simulink model "ALL_JP360_DBW_V6_5_1103"  (R2022a)
settings: Solver=FixedStepAuto  StartTime=0.0  StopTime=inf  FixedStep=0.01  RelTol=1e-3  EnableMultiTasking=on
model workspace (MAT data in the model file):
  g = 9.8
undefined symbols (not defined in the file or in its folder): canChannel, delta_v_p, IPM_Line_C0, IPM_Line_C1, IPM_Line_C2, IPM_Line_C3, M, M_p, MRR_ObjDistX, MRR_ObjDistY, MRR_ObjFusionCamID, MRR_ObjFusionSig, MRR_ObjID, MRR_ObjRelVelX, MRR_ObjRelVelY, MRR_ObjType, MRR_ObjUpdFlg, none, obj_vaild, untracktime, V, videoinput
libraries: canfdmsglib x230, canfdlib x76, slpidlib x24, simulink x18, dspstat3 x14, ctrlSharedLib x1, simulink_extras x1, imaqlib x1, realtime_pacer_lib x1, dspvision x1, visionsinks x1
(part 7 of 55)

== system ALL_JP360_DBW_V6_5_1103/MsgFromCAN/Subsystem ==
  VR_ADCU_MRR_Obj_01_02_0x690FromOutData : Inport
  VR_ADCU_MRR_Obj_03_04_0x691FromOutData : Inport  Port=2
  VR_ADCU_MRR_Obj_05_06_0x692FromOutData : Inport  Port=3
  VR_ADCU_MRR_Obj_07_08_0x693FromOutData : Inport  Port=4
  VR_ADCU_MRR_Obj_09_10_0x694FromOutData : Inport  Port=5
  VR_ADCU_MRR_Obj_11_12_0x695FromOutData : Inport  Port=6
  VR_ADCU_MRR_Obj_13_14_0x696FromOutData : Inport  Port=7
  VR_ADCU_MRR_Obj_15_16_0x697FromOutData : Inport  Port=8
  VR_ADCU_MRR_Obj_17_18_0x698FromOutData : Inport  Port=9
  VR_ADCU_MRR_Obj_19_20_0x699FromOutData : Inport  Port=10
  VR_ADCU_MRR_Obj_21_22_0x69AFromOutData : Inport  Port=11
  VR_ADCU_MRR_Obj_23_24_0x69BFromOutData : Inport  Port=12
  VR_ADCU_MRR_Obj_25_26_0x69CFromOutData : Inport  Port=13
  VR_ADCU_MRR_Obj_27_28_0x69DFromOutData : Inport  Port=14
  VR_ADCU_MRR_Obj_29_30_0x69EFromOutData : Inport  Port=15
  VR_ADCU_MRR_Obj_31_32_0x69FFromOutData : Inport  Port=16
  Subsystem1 : Subsystem
  Subsystem10 : Subsystem
  Subsystem11 : Subsystem
  Subsystem12 : Subsystem
  Subsystem13 : Subsystem
  Subsystem14 : Subsystem
  Subsystem15 : Subsystem
  Subsystem16 : Subsystem
  Subsystem2 : Subsystem
  Subsystem3 : Subsystem
  Subsystem4 : Subsystem
  Subsystem5 : Subsystem
  Subsystem6 : Subsystem
  Subsystem7 : Subsystem
  Subsystem8 : Subsystem
  Subsystem9 : Subsystem
  1 : Outport
  2 : Outport  Port=2
  3 : Outport  Port=3
  4 : Outport  Port=4
  5 : Outport  Port=5
  6 : Outport  Port=6
  7 : Outport  Port=7
  8 : Outport  Port=8
  9 : Outport  Port=9
  10 : Outport  Port=10
  11 : Outport  Port=11
  12 : Outport  Port=12
  13 : Outport  Port=13
  14 : Outport  Port=14
  15 : Outport  Port=15
  16 : Outport  Port=16
  17 : Outport  Port=17
  18 : Outport  Port=18
  19 : Outport  Port=19
  20 : Outport  Port=20
  21 : Outport  Port=21
  22 : Outport  Port=22
  23 : Outport  Port=23
  24 : Outport  Port=24
  25 : Outport  Port=25
  26 : Outport  Port=26
  27 : Outport  Port=27
  28 : Outport  Port=28
  29 : Outport  Port=29
  30 : Outport  Port=30
  31 : Outport  Port=31
  32 : Outport  Port=32
  wires:
  VR_ADCU_MRR_Obj_01_02_0x690FromOutData/1 -> Subsystem16/1(VR_ADCU_MRR_ObjHeader_0x680FromOutData)  "VR_ADCU_MRR_ObjHeader_0x680FromOutData"
  Subsystem16/1(Out1) -> 1/1
  Subsystem16/2(Out2) -> 2/1
  Subsystem1/2(Out2) -> 4/1
  Subsystem1/1(Out1) -> 3/1
  VR_ADCU_MRR_Obj_03_04_0x691FromOutData/1 -> Subsystem1/1(VR_ADCU_MRR_ObjHeader_0x680FromOutData)  "VR_ADCU_MRR_ObjHeader_0x680FromOutData"
  Subsystem3/1(Out1) -> 7/1
  Subsystem3/2(Out2) -> 8/1
  Subsystem2/2(Out2) -> 6/1
  Subsystem2/1(Out1) -> 5/1
  VR_ADCU_MRR_Obj_05_06_0x692FromOutData/1 -> Subsystem2/1(VR_ADCU_MRR_ObjHeader_0x680FromOutData)
  VR_ADCU_MRR_Obj_07_08_0x693FromOutData/1 -> Subsystem3/1(VR_ADCU_MRR_ObjHeader_0x680FromOutData)
  Subsystem6/1(Out1) -> 13/1
  Subsystem6/2(Out2) -> 14/1
  Subsystem7/2(Out2) -> 16/1
  Subsystem7/1(Out1) -> 15/1
  Subsystem5/1(Out1) -> 11/1
  Subsystem5/2(Out2) -> 12/1
  Subsystem4/2(Out2) -> 10/1
  Subsystem4/1(Out1) -> 9/1
  Subsystem12/1(Out1) -> 25/1
  Subsystem12/2(Out2) -> 26/1
  Subsystem13/2(Out2) -> 28/1
  Subsystem13/1(Out1) -> 27/1
  Subsystem15/1(Out1) -> 31/1
  Subsystem15/2(Out2) -> 32/1
  Subsystem14/2(Out2) -> 30/1
  Subsystem14/1(Out1) -> 29/1
  Subsystem10/1(Out1) -> 21/1
  Subsystem10/2(Out2) -> 22/1
  Subsystem11/2(Out2) -> 24/1
  Subsystem11/1(Out1) -> 23/1
  Subsystem9/1(Out1) -> 19/1
  Subsystem9/2(Out2) -> 20/1
  Subsystem8/2(Out2) -> 18/1
  Subsystem8/1(Out1) -> 17/1
  VR_ADCU_MRR_Obj_09_10_0x694FromOutData/1 -> Subsystem4/1(VR_ADCU_MRR_ObjHeader_0x680FromOutData)
  VR_ADCU_MRR_Obj_11_12_0x695FromOutData/1 -> Subsystem5/1(VR_ADCU_MRR_ObjHeader_0x680FromOutData)
  VR_ADCU_MRR_Obj_13_14_0x696FromOutData/1 -> Subsystem6/1(VR_ADCU_MRR_ObjHeader_0x680FromOutData)
  VR_ADCU_MRR_Obj_15_16_0x697FromOutData/1 -> Subsystem7/1(VR_ADCU_MRR_ObjHeader_0x680FromOutData)
  VR_ADCU_MRR_Obj_17_18_0x698FromOutData/1 -> Subsystem8/1(VR_ADCU_MRR_ObjHeader_0x680FromOutData)
  VR_ADCU_MRR_Obj_19_20_0x699FromOutData/1 -> Subsystem9/1(VR_ADCU_MRR_ObjHeader_0x680FromOutData)
  VR_ADCU_MRR_Obj_21_22_0x69AFromOutData/1 -> Subsystem10/1(VR_ADCU_MRR_ObjHeader_0x680FromOutData)
  VR_ADCU_MRR_Obj_23_24_0x69BFromOutData/1 -> Subsystem11/1(VR_ADCU_MRR_ObjHeader_0x680FromOutData)
  VR_ADCU_MRR_Obj_25_26_0x69CFromOutData/1 -> Subsystem12/1(VR_ADCU_MRR_ObjHeader_0x680FromOutData)
  VR_ADCU_MRR_Obj_27_28_0x69DFromOutData/1 -> Subsystem13/1(VR_ADCU_MRR_ObjHeader_0x680FromOutData)
  VR_ADCU_MRR_Obj_29_30_0x69EFromOutData/1 -> Subsystem14/1(VR_ADCU_MRR_ObjHeader_0x680FromOutData)
  VR_ADCU_MRR_Obj_31_32_0x69FFromOutData/1 -> Subsystem15/1(VR_ADCU_MRR_ObjHeader_0x680FromOutData)

== system ALL_JP360_DBW_V6_5_1103/MsgFromCAN/Subsystem1 ==
  VR_ADCU_IPM_Obj_01_0x650FromOutData : Inport
  VR_ADCU_IPM_Obj_02_0x651FromOutData : Inport  Port=2
  VR_ADCU_IPM_Obj_03_0x652FromOutData : Inport  Port=3
  VR_ADCU_IPM_Obj_04_0x653FromOutData : Inport  Port=4
  VR_ADCU_IPM_Obj_05_0x654FromOutData : Inport  Port=5
  VR_ADCU_IPM_Obj_06_0x655FromOutData : Inport  Port=6
  VR_ADCU_IPM_Obj_07_0x656FromOutData : Inport  Port=7
  VR_ADCU_IPM_Obj_08_0x657FromOutData : Inport  Port=8
  VR_ADCU_IPM_Obj_09_0x658FromOutData : Inport  Port=9
  VR_ADCU_IPM_Obj_10_0x659FromOutData : Inport  Port=10
  VR_ADCU_IPM_Obj_11_0x65AFromOutData : Inport  Port=11
  VR_ADCU_IPM_Obj_12_0x65BFromOutData : Inport  Port=12
  VR_ADCU_IPM_Obj_13_0x65CFromOutData : Inport  Port=13
  VR_ADCU_IPM_Obj_14_0x65DFromOutData : Inport  Port=14
  VR_ADCU_IPM_Obj_15_0x65EFromOutData : Inport  Port=15
  VR_ADCU_IPM_Obj_16_0x65FFromOutData : Inport  Port=16
  VR_ADCU_IPM_Obj_17_0x660FromOutData : Inport  Port=17
  VR_ADCU_IPM_Obj_18_0x661FromOutData : Inport  Port=18
  VR_ADCU_IPM_Obj_19_0x662FromOutData : Inport  Port=19
  VR_ADCU_IPM_Obj_20_0x663FromOutData : Inport  Port=20
  Subsystem1 : Subsystem
  Subsystem10 : Subsystem
  Subsystem11 : Subsystem
  Subsystem12 : Subsystem
  Subsystem13 : Subsystem
  Subsystem14 : Subsystem
  Subsystem15 : Subsystem
  Subsystem16 : Subsystem
  Subsystem17 : Subsystem
  Subsystem18 : Subsystem
  Subsystem19 : Subsystem
  Subsystem2 : Subsystem
  Subsystem20 : Subsystem
  Subsystem3 : Subsystem
  Subsystem4 : Subsystem
  Subsystem5 : Subsystem
  Subsystem6 : Subsystem
  Subsystem7 : Subsystem
  Subsystem8 : Subsystem
  Subsystem9 : Subsystem
  1 : Outport
  2 : Outport  Port=2
  3 : Outport  Port=3
  4 : Outport  Port=4
  5 : Outport  Port=5
  6 : Outport  Port=6
  7 : Outport  Port=7
  8 : Outport  Port=8
  9 : Outport  Port=9
  10 : Outport  Port=10
  11 : Outport  Port=11
  12 : Outport  Port=12
  13 : Outport  Port=13
  14 : Outport  Port=14
  15 : Outport  Port=15
  16 : Outport  Port=16
  17 : Outport  Port=17
  18 : Outport  Port=18
  19 : Outport  Port=19
  20 : Outport  Port=20
  wires:
  VR_ADCU_IPM_Obj_01_0x650FromOutData/1 -> Subsystem7/1(VR_ADCU_MRR_ObjHeader_0x680FromOutData)
  Subsystem7/1(Out2) -> 1/1
  Subsystem1/1(Out2) -> 2/1
  Subsystem2/1(Out2) -> 3/1
  Subsystem3/1(Out2) -> 5/1
  Subsystem5/1(Out2) -> 4/1
  Subsystem4/1(Out2) -> 6/1
  Subsystem9/1(Out2) -> 7/1
  Subsystem6/1(Out2) -> 8/1
  Subsystem8/1(Out2) -> 9/1
  Subsystem10/1(Out2) -> 11/1
  Subsystem16/1(Out2) -> 10/1
  Subsystem15/1(Out2) -> 17/1
  Subsystem18/1(Out2) -> 16/1
  Subsystem17/1(Out2) -> 18/1
  Subsystem11/1(Out2) -> 12/1
  Subsystem12/1(Out2) -> 14/1
  Subsystem14/1(Out2) -> 13/1
  Subsystem13/1(Out2) -> 15/1
  Subsystem20/1(Out2) -> 20/1
  Subsystem19/1(Out2) -> 19/1
  VR_ADCU_IPM_Obj_02_0x651FromOutData/1 -> Subsystem1/1(VR_ADCU_MRR_ObjHeader_0x680FromOutData)
  VR_ADCU_IPM_Obj_03_0x652FromOutData/1 -> Subsystem2/1(VR_ADCU_MRR_ObjHeader_0x680FromOutData)
  VR_ADCU_IPM_Obj_04_0x653FromOutData/1 -> Subsystem5/1(VR_ADCU_MRR_ObjHeader_0x680FromOutData)
  VR_ADCU_IPM_Obj_05_0x654FromOutData/1 -> Subsystem3/1(VR_ADCU_MRR_ObjHeader_0x680FromOutData)
  VR_ADCU_IPM_Obj_06_0x655FromOutData/1 -> Subsystem4/1(VR_ADCU_MRR_ObjHeader_0x680FromOutData)
  VR_ADCU_IPM_Obj_07_0x656FromOutData/1 -> Subsystem9/1(VR_ADCU_MRR_ObjHeader_0x680FromOutData)
  VR_ADCU_IPM_Obj_08_0x657FromOutData/1 -> Subsystem6/1(VR_ADCU_MRR_ObjHeader_0x680FromOutData)
  VR_ADCU_IPM_Obj_09_0x658FromOutData/1 -> Subsystem8/1(VR_ADCU_MRR_ObjHeader_0x680FromOutData)
  VR_ADCU_IPM_Obj_10_0x659FromOutData/1 -> Subsystem16/1(VR_ADCU_MRR_ObjHeader_0x680FromOutData)
  VR_ADCU_IPM_Obj_11_0x65AFromOutData/1 -> Subsystem10/1(VR_ADCU_MRR_ObjHeader_0x680FromOutData)
  VR_ADCU_IPM_Obj_12_0x65BFromOutData/1 -> Subsystem11/1(VR_ADCU_MRR_ObjHeader_0x680FromOutData)
  VR_ADCU_IPM_Obj_13_0x65CFromOutData/1 -> Subsystem14/1(VR_ADCU_MRR_ObjHeader_0x680FromOutData)
  VR_ADCU_IPM_Obj_14_0x65DFromOutData/1 -> Subsystem12/1(VR_ADCU_MRR_ObjHeader_0x680FromOutData)
  VR_ADCU_IPM_Obj_15_0x65EFromOutData/1 -> Subsystem13/1(VR_ADCU_MRR_ObjHeader_0x680FromOutData)
  VR_ADCU_IPM_Obj_16_0x65FFromOutData/1 -> Subsystem18/1(VR_ADCU_MRR_ObjHeader_0x680FromOutData)
  VR_ADCU_IPM_Obj_17_0x660FromOutData/1 -> Subsystem15/1(VR_ADCU_MRR_ObjHeader_0x680FromOutData)
  VR_ADCU_IPM_Obj_18_0x661FromOutData/1 -> Subsystem17/1(VR_ADCU_MRR_ObjHeader_0x680FromOutData)
  VR_ADCU_IPM_Obj_19_0x662FromOutData/1 -> Subsystem19/1(VR_ADCU_MRR_ObjHeader_0x680FromOutData)
  VR_ADCU_IPM_Obj_20_0x663FromOutData/1 -> Subsystem20/1(VR_ADCU_MRR_ObjHeader_0x680FromOutData)

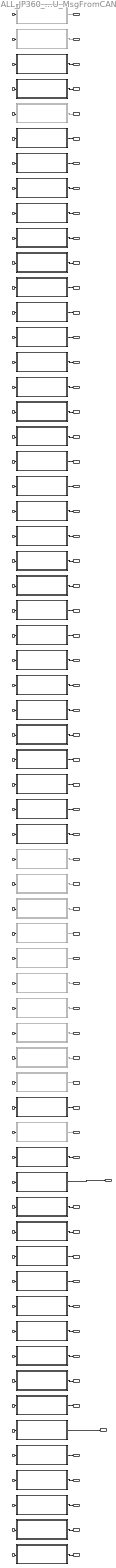
== system ALL_JP360_DBW_V6_5_1103/MsgFromCAN/VR_ADCU_MsgFromCAN ==
  VR_ADCU_IPM_0x345FromInData : Inport  OutDataTypeStr=Bus:CAN_FD_MESSAGE_BUS
  VR_ADCU_IPM_0x347FromInData : Inport  Port=2  OutDataTypeStr=Bus:CAN_FD_MESSAGE_BUS
  VR_ADCU_IPM_LeftLine_0x378FromInData : Inport  Port=3  OutDataTypeStr=Bus:CAN_FD_MESSAGE_BUS
  VR_ADCU_IPM_LeftLine_0x380FromInData : Inport  Port=4  OutDataTypeStr=Bus:CAN_FD_MESSAGE_BUS
  VR_ADCU_IPM_LineHeader_0x631FromInData : Inport  Port=5  OutDataTypeStr=Bus:CAN_FD_MESSAGE_BUS
  VR_ADCU_IPM_Line_01_0x640FromInData : Inport  Port=6  OutDataTypeStr=Bus:CAN_FD_MESSAGE_BUS
  VR_ADCU_IPM_Line_02_0x641FromInData : Inport  Port=7  OutDataTypeStr=Bus:CAN_FD_MESSAGE_BUS
  VR_ADCU_IPM_Line_03_0x642FromInData : Inport  Port=8  OutDataTypeStr=Bus:CAN_FD_MESSAGE_BUS
  VR_ADCU_IPM_Line_04_0x643FromInData : Inport  Port=9  OutDataTypeStr=Bus:CAN_FD_MESSAGE_BUS
  VR_ADCU_IPM_Line_05_0x644FromInData : Inport  Port=10  OutDataTypeStr=Bus:CAN_FD_MESSAGE_BUS
  VR_ADCU_IPM_Line_06_0x645FromInData : Inport  Port=11  OutDataTypeStr=Bus:CAN_FD_MESSAGE_BUS
  VR_ADCU_IPM_ObjHeader_0x630FromInData : Inport  Port=12  OutDataTypeStr=Bus:CAN_FD_MESSAGE_BUS
  VR_ADCU_IPM_Obj_01_0x650FromInData : Inport  Port=13  OutDataTypeStr=Bus:CAN_FD_MESSAGE_BUS
  VR_ADCU_IPM_Obj_02_0x651FromInData : Inport  Port=14  OutDataTypeStr=Bus:CAN_FD_MESSAGE_BUS
  VR_ADCU_IPM_Obj_03_0x652FromInData : Inport  Port=15  OutDataTypeStr=Bus:CAN_FD_MESSAGE_BUS
  VR_ADCU_IPM_Obj_04_0x653FromInData : Inport  Port=16  OutDataTypeStr=Bus:CAN_FD_MESSAGE_BUS
  VR_ADCU_IPM_Obj_05_0x654FromInData : Inport  Port=17  OutDataTypeStr=Bus:CAN_FD_MESSAGE_BUS
  VR_ADCU_IPM_Obj_06_0x655FromInData : Inport  Port=18  OutDataTypeStr=Bus:CAN_FD_MESSAGE_BUS
  VR_ADCU_IPM_Obj_07_0x656FromInData : Inport  Port=19  OutDataTypeStr=Bus:CAN_FD_MESSAGE_BUS
  VR_ADCU_IPM_Obj_08_0x657FromInData : Inport  Port=20  OutDataTypeStr=Bus:CAN_FD_MESSAGE_BUS
  VR_ADCU_IPM_Obj_09_0x658FromInData : Inport  Port=21  OutDataTypeStr=Bus:CAN_FD_MESSAGE_BUS
  VR_ADCU_IPM_Obj_10_0x659FromInData : Inport  Port=22  OutDataTypeStr=Bus:CAN_FD_MESSAGE_BUS
  VR_ADCU_IPM_Obj_11_0x65AFromInData : Inport  Port=23  OutDataTypeStr=Bus:CAN_FD_MESSAGE_BUS
  VR_ADCU_IPM_Obj_12_0x65BFromInData : Inport  Port=24  OutDataTypeStr=Bus:CAN_FD_MESSAGE_BUS
  VR_ADCU_IPM_Obj_13_0x65CFromInData : Inport  Port=25  OutDataTypeStr=Bus:CAN_FD_MESSAGE_BUS
  VR_ADCU_IPM_Obj_14_0x65DFromInData : Inport  Port=26  OutDataTypeStr=Bus:CAN_FD_MESSAGE_BUS
  VR_ADCU_IPM_Obj_15_0x65EFromInData : Inport  Port=27  OutDataTypeStr=Bus:CAN_FD_MESSAGE_BUS
  VR_ADCU_IPM_Obj_16_0x65FFromInData : Inport  Port=28  OutDataTypeStr=Bus:CAN_FD_MESSAGE_BUS
  VR_ADCU_IPM_Obj_17_0x660FromInData : Inport  Port=29  OutDataTypeStr=Bus:CAN_FD_MESSAGE_BUS
  VR_ADCU_IPM_Obj_18_0x661FromInData : Inport  Port=30  OutDataTypeStr=Bus:CAN_FD_MESSAGE_BUS
  VR_ADCU_IPM_Obj_19_0x662FromInData : Inport  Port=31  OutDataTypeStr=Bus:CAN_FD_MESSAGE_BUS
  VR_ADCU_IPM_Obj_20_0x663FromInData : Inport  Port=32  OutDataTypeStr=Bus:CAN_FD_MESSAGE_BUS
  VR_ADCU_IPM_RightLine_0x590FromInData : Inport  Port=33  OutDataTypeStr=Bus:CAN_FD_MESSAGE_BUS
  VR_ADCU_IPM_RightLine_0x591FromInData : Inport  Port=34  OutDataTypeStr=Bus:CAN_FD_MESSAGE_BUS
  VR_ADCU_IPM_Traffic_01_0x670FromInData : Inport  Port=35  OutDataTypeStr=Bus:CAN_FD_MESSAGE_BUS
  VR_ADCU_IPM_Traffic_02_0x671FromInData : Inport  Port=36  OutDataTypeStr=Bus:CAN_FD_MESSAGE_BUS
  VR_ADCU_IPM_Traffic_03_0x672FromInData : Inport  Port=37  OutDataTypeStr=Bus:CAN_FD_MESSAGE_BUS
  VR_ADCU_IPM_Traffic_04_0x673FromInData : Inport  Port=38  OutDataTypeStr=Bus:CAN_FD_MESSAGE_BUS
  VR_ADCU_IPM_Traffic_05_0x674FromInData : Inport  Port=39  OutDataTypeStr=Bus:CAN_FD_MESSAGE_BUS
  VR_ADCU_IPM_Traffic_06_0x675FromInData : Inport  Port=40  OutDataTypeStr=Bus:CAN_FD_MESSAGE_BUS
  VR_ADCU_IPM_VLC_0x393FromInData : Inport  Port=41  OutDataTypeStr=Bus:CAN_FD_MESSAGE_BUS
  VR_ADCU_MRR_0x338FromInData : Inport  Port=42  OutDataTypeStr=Bus:CAN_FD_MESSAGE_BUS
  VR_ADCU_MRR_0x339FromInData : Inport  Port=43  OutDataTypeStr=Bus:CAN_FD_MESSAGE_BUS
  VR_ADCU_MRR_0x346FromInData : Inport  Port=44  OutDataTypeStr=Bus:CAN_FD_MESSAGE_BUS
  VR_ADCU_MRR_FRObj_0x379FromInData : Inport  Port=45  OutDataTypeStr=Bus:CAN_FD_MESSAGE_BUS
  VR_ADCU_MRR_LRObj_0x580FromInData : Inport  Port=46  OutDataTypeStr=Bus:CAN_FD_MESSAGE_BUS
  VR_ADCU_MRR_ObjHeader_0x680FromInData : Inport  Port=47  OutDataTypeStr=Bus:CAN_FD_MESSAGE_BUS
  VR_ADCU_MRR_Obj_01_02_0x690FromInData : Inport  Port=48  OutDataTypeStr=Bus:CAN_FD_MESSAGE_BUS
  VR_ADCU_MRR_Obj_03_04_0x691FromInData : Inport  Port=49  OutDataTypeStr=Bus:CAN_FD_MESSAGE_BUS
  VR_ADCU_MRR_Obj_05_06_0x692FromInData : Inport  Port=50  OutDataTypeStr=Bus:CAN_FD_MESSAGE_BUS
  VR_ADCU_MRR_Obj_07_08_0x693FromInData : Inport  Port=51  OutDataTypeStr=Bus:CAN_FD_MESSAGE_BUS
  VR_ADCU_MRR_Obj_09_10_0x694FromInData : Inport  Port=52  OutDataTypeStr=Bus:CAN_FD_MESSAGE_BUS
  VR_ADCU_MRR_Obj_11_12_0x695FromInData : Inport  Port=53  OutDataTypeStr=Bus:CAN_FD_MESSAGE_BUS
  VR_ADCU_MRR_Obj_13_14_0x696FromInData : Inport  Port=54  OutDataTypeStr=Bus:CAN_FD_MESSAGE_BUS
  VR_ADCU_MRR_Obj_15_16_0x697FromInData : Inport  Port=55  OutDataTypeStr=Bus:CAN_FD_MESSAGE_BUS
  VR_ADCU_MRR_Obj_17_18_0x698FromInData : Inport  Port=56  OutDataTypeStr=Bus:CAN_FD_MESSAGE_BUS
  VR_ADCU_MRR_Obj_19_20_0x699FromInData : Inport  Port=57  OutDataTypeStr=Bus:CAN_FD_MESSAGE_BUS
  VR_ADCU_MRR_Obj_21_22_0x69AFromInData : Inport  Port=58  OutDataTypeStr=Bus:CAN_FD_MESSAGE_BUS
  VR_ADCU_MRR_Obj_23_24_0x69BFromInData : Inport  Port=59  OutDataTypeStr=Bus:CAN_FD_MESSAGE_BUS
  VR_ADCU_MRR_Obj_25_26_0x69CFromInData : Inport  Port=60  OutDataTypeStr=Bus:CAN_FD_MESSAGE_BUS
  VR_ADCU_MRR_Obj_27_28_0x69DFromInData : Inport  Port=61  OutDataTypeStr=Bus:CAN_FD_MESSAGE_BUS
  VR_ADCU_MRR_Obj_29_30_0x69EFromInData : Inport  Port=62  OutDataTypeStr=Bus:CAN_FD_MESSAGE_BUS
  VR_ADCU_MRR_Obj_31_32_0x69FFromInData : Inport  Port=63  OutDataTypeStr=Bus:CAN_FD_MESSAGE_BUS
  VR_ADCU_IPM_0x345 : Subsystem  Commented=on  TreatAsAtomicUnit=on
  VR_ADCU_IPM_0x347 : Subsystem  Commented=on  TreatAsAtomicUnit=on
  VR_ADCU_IPM_LeftLine_0x378 : Subsystem  TreatAsAtomicUnit=on
  VR_ADCU_IPM_LeftLine_0x380 : Subsystem  TreatAsAtomicUnit=on
  VR_ADCU_IPM_LineHeader_0x631 : Subsystem  Commented=on  TreatAsAtomicUnit=on
  VR_ADCU_IPM_Line_01_0x640 : Subsystem  TreatAsAtomicUnit=on
  VR_ADCU_IPM_Line_02_0x641 : Subsystem  TreatAsAtomicUnit=on
  VR_ADCU_IPM_Line_03_0x642 : Subsystem  TreatAsAtomicUnit=on
  VR_ADCU_IPM_Line_04_0x643 : Subsystem  TreatAsAtomicUnit=on
  VR_ADCU_IPM_Line_05_0x644 : Subsystem  TreatAsAtomicUnit=on
  VR_ADCU_IPM_Line_06_0x645 : Subsystem  TreatAsAtomicUnit=on
  VR_ADCU_IPM_ObjHeader_0x630 : Subsystem  TreatAsAtomicUnit=on
  VR_ADCU_IPM_Obj_01_0x650 : Subsystem  TreatAsAtomicUnit=on
  VR_ADCU_IPM_Obj_02_0x651 : Subsystem  TreatAsAtomicUnit=on
  VR_ADCU_IPM_Obj_03_0x652 : Subsystem  TreatAsAtomicUnit=on
  VR_ADCU_IPM_Obj_04_0x653 : Subsystem  TreatAsAtomicUnit=on
  VR_ADCU_IPM_Obj_05_0x654 : Subsystem  TreatAsAtomicUnit=on
  VR_ADCU_IPM_Obj_06_0x655 : Subsystem  TreatAsAtomicUnit=on
  VR_ADCU_IPM_Obj_07_0x656 : Subsystem  TreatAsAtomicUnit=on
  VR_ADCU_IPM_Obj_08_0x657 : Subsystem  TreatAsAtomicUnit=on
  VR_ADCU_IPM_Obj_09_0x658 : Subsystem  TreatAsAtomicUnit=on
  VR_ADCU_IPM_Obj_10_0x659 : Subsystem  TreatAsAtomicUnit=on
  VR_ADCU_IPM_Obj_11_0x65A : Subsystem  TreatAsAtomicUnit=on
  VR_ADCU_IPM_Obj_12_0x65B : Subsystem  TreatAsAtomicUnit=on
  VR_ADCU_IPM_Obj_13_0x65C : Subsystem  TreatAsAtomicUnit=on
  VR_ADCU_IPM_Obj_14_0x65D : Subsystem  TreatAsAtomicUnit=on
  VR_ADCU_IPM_Obj_15_0x65E : Subsystem  TreatAsAtomicUnit=on
  VR_ADCU_IPM_Obj_16_0x65F : Subsystem  TreatAsAtomicUnit=on
  VR_ADCU_IPM_Obj_17_0x660 : Subsystem  TreatAsAtomicUnit=on
  VR_ADCU_IPM_Obj_18_0x661 : Subsystem  TreatAsAtomicUnit=on
  VR_ADCU_IPM_Obj_19_0x662 : Subsystem  TreatAsAtomicUnit=on
  VR_ADCU_IPM_Obj_20_0x663 : Subsystem  TreatAsAtomicUnit=on
  VR_ADCU_IPM_RightLine_0x590 : Subsystem  TreatAsAtomicUnit=on
  VR_ADCU_IPM_RightLine_0x591 : Subsystem  TreatAsAtomicUnit=on
  VR_ADCU_IPM_Traffic_01_0x670 : Subsystem  Commented=on  TreatAsAtomicUnit=on
  VR_ADCU_IPM_Traffic_02_0x671 : Subsystem  Commented=on  TreatAsAtomicUnit=on
  VR_ADCU_IPM_Traffic_03_0x672 : Subsystem  Commented=on  TreatAsAtomicUnit=on
  VR_ADCU_IPM_Traffic_04_0x673 : Subsystem  Commented=on  TreatAsAtomicUnit=on
  VR_ADCU_IPM_Traffic_05_0x674 : Subsystem  Commented=on  TreatAsAtomicUnit=on
  VR_ADCU_IPM_Traffic_06_0x675 : Subsystem  Commented=on  TreatAsAtomicUnit=on
  VR_ADCU_IPM_VLC_0x393 : Subsystem  Commented=on  TreatAsAtomicUnit=on
  VR_ADCU_MRR_0x338 : Subsystem  Commented=on  TreatAsAtomicUnit=on
  VR_ADCU_MRR_0x339 : Subsystem  Commented=on  TreatAsAtomicUnit=on
  VR_ADCU_MRR_0x346 : Subsystem  Commented=on  TreatAsAtomicUnit=on
  VR_ADCU_MRR_FRObj_0x379 : Subsystem  TreatAsAtomicUnit=on
  VR_ADCU_MRR_LRObj_0x580 : Subsystem  Commented=on  TreatAsAtomicUnit=on
  VR_ADCU_MRR_ObjHeader_0x680 : Subsystem  TreatAsAtomicUnit=on
  VR_ADCU_MRR_Obj_01_02_0x690 : Subsystem  TreatAsAtomicUnit=on
  VR_ADCU_MRR_Obj_03_04_0x691 : Subsystem  TreatAsAtomicUnit=on
  VR_ADCU_MRR_Obj_05_06_0x692 : Subsystem  TreatAsAtomicUnit=on
  VR_ADCU_MRR_Obj_07_08_0x693 : Subsystem  TreatAsAtomicUnit=on
  VR_ADCU_MRR_Obj_09_10_0x694 : Subsystem  TreatAsAtomicUnit=on
  VR_ADCU_MRR_Obj_11_12_0x695 : Subsystem  TreatAsAtomicUnit=on
  VR_ADCU_MRR_Obj_13_14_0x696 : Subsystem  TreatAsAtomicUnit=on
  VR_ADCU_MRR_Obj_15_16_0x697 : Subsystem  TreatAsAtomicUnit=on
  VR_ADCU_MRR_Obj_17_18_0x698 : Subsystem  TreatAsAtomicUnit=on
  VR_ADCU_MRR_Obj_19_20_0x699 : Subsystem  TreatAsAtomicUnit=on
  VR_ADCU_MRR_Obj_21_22_0x69A : Subsystem  TreatAsAtomicUnit=on
  VR_ADCU_MRR_Obj_23_24_0x69B : Subsystem  TreatAsAtomicUnit=on
  VR_ADCU_MRR_Obj_25_26_0x69C : Subsystem  TreatAsAtomicUnit=on
  VR_ADCU_MRR_Obj_27_28_0x69D : Subsystem  TreatAsAtomicUnit=on
  VR_ADCU_MRR_Obj_29_30_0x69E : Subsystem  TreatAsAtomicUnit=on
  VR_ADCU_MRR_Obj_31_32_0x69F : Subsystem  TreatAsAtomicUnit=on
  VR_ADCU_IPM_0x345FromOutData : Outport  OutDataTypeStr=Bus:VR_ADCU_IPM_0x345
  VR_ADCU_IPM_0x347FromOutData : Outport  Port=2  OutDataTypeStr=Bus:VR_ADCU_IPM_0x347
  VR_ADCU_IPM_LeftLine_0x378FromOutData : Outport  Port=3  OutDataTypeStr=Bus:VR_ADCU_IPM_LeftLine_0x378
  VR_ADCU_IPM_LeftLine_0x380FromOutData : Outport  Port=4  OutDataTypeStr=Bus:VR_ADCU_IPM_LeftLine_0x380
  VR_ADCU_IPM_LineHeader_0x631FromOutData : Outport  Port=5  OutDataTypeStr=Bus:VR_ADCU_IPM_LineHeader_0x631
  VR_ADCU_IPM_Line_01_0x640FromOutData : Outport  Port=6  OutDataTypeStr=Bus:VR_ADCU_IPM_Line_01_0x640
  VR_ADCU_IPM_Line_02_0x641FromOutData : Outport  Port=7  OutDataTypeStr=Bus:VR_ADCU_IPM_Line_02_0x641
  VR_ADCU_IPM_Line_03_0x642FromOutData : Outport  Port=8  OutDataTypeStr=Bus:VR_ADCU_IPM_Line_03_0x642
  VR_ADCU_IPM_Line_04_0x643FromOutData : Outport  Port=9  OutDataTypeStr=Bus:VR_ADCU_IPM_Line_04_0x643
  VR_ADCU_IPM_Line_05_0x644FromOutData : Outport  Port=10  OutDataTypeStr=Bus:VR_ADCU_IPM_Line_05_0x644
  VR_ADCU_IPM_Line_06_0x645FromOutData : Outport  Port=11  OutDataTypeStr=Bus:VR_ADCU_IPM_Line_06_0x645
  VR_ADCU_IPM_ObjHeader_0x630FromOutData : Outport  Port=12  OutDataTypeStr=Bus:VR_ADCU_IPM_ObjHeader_0x630
  VR_ADCU_IPM_Obj_01_0x650FromOutData : Outport  Port=13  OutDataTypeStr=Bus:VR_ADCU_IPM_Obj_01_0x650
  VR_ADCU_IPM_Obj_02_0x651FromOutData : Outport  Port=14  OutDataTypeStr=Bus:VR_ADCU_IPM_Obj_02_0x651
  VR_ADCU_IPM_Obj_03_0x652FromOutData : Outport  Port=15  OutDataTypeStr=Bus:VR_ADCU_IPM_Obj_03_0x652
  VR_ADCU_IPM_Obj_04_0x653FromOutData : Outport  Port=16  OutDataTypeStr=Bus:VR_ADCU_IPM_Obj_04_0x653
  VR_ADCU_IPM_Obj_05_0x654FromOutData : Outport  Port=17  OutDataTypeStr=Bus:VR_ADCU_IPM_Obj_05_0x654
  VR_ADCU_IPM_Obj_06_0x655FromOutData : Outport  Port=18  OutDataTypeStr=Bus:VR_ADCU_IPM_Obj_06_0x655
  VR_ADCU_IPM_Obj_07_0x656FromOutData : Outport  Port=19  OutDataTypeStr=Bus:VR_ADCU_IPM_Obj_07_0x656
  VR_ADCU_IPM_Obj_08_0x657FromOutData : Outport  Port=20  OutDataTypeStr=Bus:VR_ADCU_IPM_Obj_08_0x657
  VR_ADCU_IPM_Obj_09_0x658FromOutData : Outport  Port=21  OutDataTypeStr=Bus:VR_ADCU_IPM_Obj_09_0x658
  VR_ADCU_IPM_Obj_10_0x659FromOutData : Outport  Port=22  OutDataTypeStr=Bus:VR_ADCU_IPM_Obj_10_0x659
  VR_ADCU_IPM_Obj_11_0x65AFromOutData : Outport  Port=23  OutDataTypeStr=Bus:VR_ADCU_IPM_Obj_11_0x65A
  VR_ADCU_IPM_Obj_12_0x65BFromOutData : Outport  Port=24  OutDataTypeStr=Bus:VR_ADCU_IPM_Obj_12_0x65B
  VR_ADCU_IPM_Obj_13_0x65CFromOutData : Outport  Port=25  OutDataTypeStr=Bus:VR_ADCU_IPM_Obj_13_0x65C
  VR_ADCU_IPM_Obj_14_0x65DFromOutData : Outport  Port=26  OutDataTypeStr=Bus:VR_ADCU_IPM_Obj_14_0x65D
  VR_ADCU_IPM_Obj_15_0x65EFromOutData : Outport  Port=27  OutDataTypeStr=Bus:VR_ADCU_IPM_Obj_15_0x65E
  VR_ADCU_IPM_Obj_16_0x65FFromOutData : Outport  Port=28  OutDataTypeStr=Bus:VR_ADCU_IPM_Obj_16_0x65F
  VR_ADCU_IPM_Obj_17_0x660FromOutData : Outport  Port=29  OutDataTypeStr=Bus:VR_ADCU_IPM_Obj_17_0x660
  VR_ADCU_IPM_Obj_18_0x661FromOutData : Outport  Port=30  OutDataTypeStr=Bus:VR_ADCU_IPM_Obj_18_0x661
  VR_ADCU_IPM_Obj_19_0x662FromOutData : Outport  Port=31  OutDataTypeStr=Bus:VR_ADCU_IPM_Obj_19_0x662
  VR_ADCU_IPM_Obj_20_0x663FromOutData : Outport  Port=32  OutDataTypeStr=Bus:VR_ADCU_IPM_Obj_20_0x663
  VR_ADCU_IPM_RightLine_0x590FromOutData : Outport  Port=33  OutDataTypeStr=Bus:VR_ADCU_IPM_RightLine_0x590
  VR_ADCU_IPM_RightLine_0x591FromOutData : Outport  Port=34  OutDataTypeStr=Bus:VR_ADCU_IPM_RightLine_0x591
  VR_ADCU_IPM_Traffic_01_0x670FromOutData : Outport  Port=35  OutDataTypeStr=Bus:VR_ADCU_IPM_Traffic_01_0x670
  VR_ADCU_IPM_Traffic_02_0x671FromOutData : Outport  Port=36  OutDataTypeStr=Bus:VR_ADCU_IPM_Traffic_02_0x671
  VR_ADCU_IPM_Traffic_03_0x672FromOutData : Outport  Port=37  OutDataTypeStr=Bus:VR_ADCU_IPM_Traffic_03_0x672
  VR_ADCU_IPM_Traffic_04_0x673FromOutData : Outport  Port=38  OutDataTypeStr=Bus:VR_ADCU_IPM_Traffic_04_0x673
  VR_ADCU_IPM_Traffic_05_0x674FromOutData : Outport  Port=39  OutDataTypeStr=Bus:VR_ADCU_IPM_Traffic_05_0x674
  VR_ADCU_IPM_Traffic_06_0x675FromOutData : Outport  Port=40  OutDataTypeStr=Bus:VR_ADCU_IPM_Traffic_06_0x675
  VR_ADCU_IPM_VLC_0x393FromOutData : Outport  Port=41  OutDataTypeStr=Bus:VR_ADCU_IPM_VLC_0x393
  VR_ADCU_MRR_0x338FromOutData : Outport  Port=42  OutDataTypeStr=Bus:VR_ADCU_MRR_0x338
  VR_ADCU_MRR_0x339FromOutData : Outport  Port=43  OutDataTypeStr=Bus:VR_ADCU_MRR_0x339
  VR_ADCU_MRR_0x346FromOutData : Outport  Port=44  OutDataTypeStr=Bus:VR_ADCU_MRR_0x346
  VR_ADCU_MRR_FRObj_0x379FromOutData : Outport  Port=45  OutDataTypeStr=Bus:VR_ADCU_MRR_FRObj_0x379
  VR_ADCU_MRR_LRObj_0x580FromOutData : Outport  Port=46  OutDataTypeStr=Bus:VR_ADCU_MRR_LRObj_0x580
  VR_ADCU_MRR_ObjHeader_0x680FromOutData : Outport  Port=47  OutDataTypeStr=Bus:VR_ADCU_MRR_ObjHeader_0x680
  VR_ADCU_MRR_Obj_01_02_0x690FromOutData : Outport  Port=48  OutDataTypeStr=Bus:VR_ADCU_MRR_Obj_01_02_0x690
  VR_ADCU_MRR_Obj_03_04_0x691FromOutData : Outport  Port=49  OutDataTypeStr=Bus:VR_ADCU_MRR_Obj_03_04_0x691
  VR_ADCU_MRR_Obj_05_06_0x692FromOutData : Outport  Port=50  OutDataTypeStr=Bus:VR_ADCU_MRR_Obj_05_06_0x692
  VR_ADCU_MRR_Obj_07_08_0x693FromOutData : Outport  Port=51  OutDataTypeStr=Bus:VR_ADCU_MRR_Obj_07_08_0x693
  VR_ADCU_MRR_Obj_09_10_0x694FromOutData : Outport  Port=52  OutDataTypeStr=Bus:VR_ADCU_MRR_Obj_09_10_0x694
  VR_ADCU_MRR_Obj_11_12_0x695FromOutData : Outport  Port=53  OutDataTypeStr=Bus:VR_ADCU_MRR_Obj_11_12_0x695
  VR_ADCU_MRR_Obj_13_14_0x696FromOutData : Outport  Port=54  OutDataTypeStr=Bus:VR_ADCU_MRR_Obj_13_14_0x696
  VR_ADCU_MRR_Obj_15_16_0x697FromOutData : Outport  Port=55  OutDataTypeStr=Bus:VR_ADCU_MRR_Obj_15_16_0x697
  VR_ADCU_MRR_Obj_17_18_0x698FromOutData : Outport  Port=56  OutDataTypeStr=Bus:VR_ADCU_MRR_Obj_17_18_0x698
  VR_ADCU_MRR_Obj_19_20_0x699FromOutData : Outport  Port=57  OutDataTypeStr=Bus:VR_ADCU_MRR_Obj_19_20_0x699
  VR_ADCU_MRR_Obj_21_22_0x69AFromOutData : Outport  Port=58  OutDataTypeStr=Bus:VR_ADCU_MRR_Obj_21_22_0x69A
  VR_ADCU_MRR_Obj_23_24_0x69BFromOutData : Outport  Port=59  OutDataTypeStr=Bus:VR_ADCU_MRR_Obj_23_24_0x69B
  VR_ADCU_MRR_Obj_25_26_0x69CFromOutData : Outport  Port=60  OutDataTypeStr=Bus:VR_ADCU_MRR_Obj_25_26_0x69C
  VR_ADCU_MRR_Obj_27_28_0x69DFromOutData : Outport  Port=61  OutDataTypeStr=Bus:VR_ADCU_MRR_Obj_27_28_0x69D
  VR_ADCU_MRR_Obj_29_30_0x69EFromOutData : Outport  Port=62  OutDataTypeStr=Bus:VR_ADCU_MRR_Obj_29_30_0x69E
  VR_ADCU_MRR_Obj_31_32_0x69FFromOutData : Outport  Port=63  OutDataTypeStr=Bus:VR_ADCU_MRR_Obj_31_32_0x69F
  wires:
  VR_ADCU_IPM_0x345/1(VR_ADCU_IPM_0x345FromOutData) -> VR_ADCU_IPM_0x345FromOutData/1  "VR_ADCU_IPM_0x345FromOutData"
  VR_ADCU_IPM_0x345FromInData/1 -> VR_ADCU_IPM_0x345/1(VR_ADCU_IPM_0x345FromInData)  "VR_ADCU_IPM_0x345FromInData"
  VR_ADCU_IPM_0x347/1(VR_ADCU_IPM_0x347FromOutData) -> VR_ADCU_IPM_0x347FromOutData/1  "VR_ADCU_IPM_0x347FromOutData"
  VR_ADCU_IPM_0x347FromInData/1 -> VR_ADCU_IPM_0x347/1(VR_ADCU_IPM_0x347FromInData)  "VR_ADCU_IPM_0x347FromInData"
  VR_ADCU_IPM_LeftLine_0x378/1(VR_ADCU_IPM_LeftLine_0x378FromOutData) -> VR_ADCU_IPM_LeftLine_0x378FromOutData/1  "VR_ADCU_IPM_LeftLine_0x378FromOutData"
  VR_ADCU_IPM_LeftLine_0x378FromInData/1 -> VR_ADCU_IPM_LeftLine_0x378/1(VR_ADCU_IPM_LeftLine_0x378FromInData)  "VR_ADCU_IPM_LeftLine_0x378FromInData"
  VR_ADCU_IPM_LeftLine_0x380/1(VR_ADCU_IPM_LeftLine_0x380FromOutData) -> VR_ADCU_IPM_LeftLine_0x380FromOutData/1  "VR_ADCU_IPM_LeftLine_0x380FromOutData"
  VR_ADCU_IPM_LeftLine_0x380FromInData/1 -> VR_ADCU_IPM_LeftLine_0x380/1(VR_ADCU_IPM_LeftLine_0x380FromInData)  "VR_ADCU_IPM_LeftLine_0x380FromInData"
  VR_ADCU_IPM_LineHeader_0x631/1(VR_ADCU_IPM_LineHeader_0x631FromOutData) -> VR_ADCU_IPM_LineHeader_0x631FromOutData/1  "VR_ADCU_IPM_LineHeader_0x631FromOutData"
  VR_ADCU_IPM_LineHeader_0x631FromInData/1 -> VR_ADCU_IPM_LineHeader_0x631/1(VR_ADCU_IPM_LineHeader_0x631FromInData)  "VR_ADCU_IPM_LineHeader_0x631FromInData"
  VR_ADCU_IPM_Line_01_0x640/1(VR_ADCU_IPM_Line_01_0x640FromOutData) -> VR_ADCU_IPM_Line_01_0x640FromOutData/1  "VR_ADCU_IPM_Line_01_0x640FromOutData"
  VR_ADCU_IPM_Line_01_0x640FromInData/1 -> VR_ADCU_IPM_Line_01_0x640/1(VR_ADCU_IPM_Line_01_0x640FromInData)  "VR_ADCU_IPM_Line_01_0x640FromInData"
  VR_ADCU_IPM_Line_02_0x641/1(VR_ADCU_IPM_Line_02_0x641FromOutData) -> VR_ADCU_IPM_Line_02_0x641FromOutData/1  "VR_ADCU_IPM_Line_02_0x641FromOutData"
  VR_ADCU_IPM_Line_02_0x641FromInData/1 -> VR_ADCU_IPM_Line_02_0x641/1(VR_ADCU_IPM_Line_02_0x641FromInData)  "VR_ADCU_IPM_Line_02_0x641FromInData"
  VR_ADCU_IPM_Line_03_0x642/1(VR_ADCU_IPM_Line_03_0x642FromOutData) -> VR_ADCU_IPM_Line_03_0x642FromOutData/1  "VR_ADCU_IPM_Line_03_0x642FromOutData"
  VR_ADCU_IPM_Line_03_0x642FromInData/1 -> VR_ADCU_IPM_Line_03_0x642/1(VR_ADCU_IPM_Line_03_0x642FromInData)  "VR_ADCU_IPM_Line_03_0x642FromInData"
  VR_ADCU_IPM_Line_04_0x643/1(VR_ADCU_IPM_Line_04_0x643FromOutData) -> VR_ADCU_IPM_Line_04_0x643FromOutData/1  "VR_ADCU_IPM_Line_04_0x643FromOutData"
  VR_ADCU_IPM_Line_04_0x643FromInData/1 -> VR_ADCU_IPM_Line_04_0x643/1(VR_ADCU_IPM_Line_04_0x643FromInData)  "VR_ADCU_IPM_Line_04_0x643FromInData"
  VR_ADCU_IPM_Line_05_0x644/1(VR_ADCU_IPM_Line_05_0x644FromOutData) -> VR_ADCU_IPM_Line_05_0x644FromOutData/1  "VR_ADCU_IPM_Line_05_0x644FromOutData"
  VR_ADCU_IPM_Line_05_0x644FromInData/1 -> VR_ADCU_IPM_Line_05_0x644/1(VR_ADCU_IPM_Line_05_0x644FromInData)  "VR_ADCU_IPM_Line_05_0x644FromInData"
  VR_ADCU_IPM_Line_06_0x645/1(VR_ADCU_IPM_Line_06_0x645FromOutData) -> VR_ADCU_IPM_Line_06_0x645FromOutData/1  "VR_ADCU_IPM_Line_06_0x645FromOutData"
  VR_ADCU_IPM_Line_06_0x645FromInData/1 -> VR_ADCU_IPM_Line_06_0x645/1(VR_ADCU_IPM_Line_06_0x645FromInData)  "VR_ADCU_IPM_Line_06_0x645FromInData"
  VR_ADCU_IPM_ObjHeader_0x630/1(VR_ADCU_IPM_ObjHeader_0x630FromOutData) -> VR_ADCU_IPM_ObjHeader_0x630FromOutData/1  "VR_ADCU_IPM_ObjHeader_0x630FromOutData"
  VR_ADCU_IPM_ObjHeader_0x630FromInData/1 -> VR_ADCU_IPM_ObjHeader_0x630/1(VR_ADCU_IPM_ObjHeader_0x630FromInData)  "VR_ADCU_IPM_ObjHeader_0x630FromInData"
  VR_ADCU_IPM_Obj_01_0x650/1(VR_ADCU_IPM_Obj_01_0x650FromOutData) -> VR_ADCU_IPM_Obj_01_0x650FromOutData/1  "VR_ADCU_IPM_Obj_01_0x650FromOutData"
  VR_ADCU_IPM_Obj_01_0x650FromInData/1 -> VR_ADCU_IPM_Obj_01_0x650/1(VR_ADCU_IPM_Obj_01_0x650FromInData)  "VR_ADCU_IPM_Obj_01_0x650FromInData"
  VR_ADCU_IPM_Obj_02_0x651/1(VR_ADCU_IPM_Obj_02_0x651FromOutData) -> VR_ADCU_IPM_Obj_02_0x651FromOutData/1  "VR_ADCU_IPM_Obj_02_0x651FromOutData"
  VR_ADCU_IPM_Obj_02_0x651FromInData/1 -> VR_ADCU_IPM_Obj_02_0x651/1(VR_ADCU_IPM_Obj_02_0x651FromInData)  "VR_ADCU_IPM_Obj_02_0x651FromInData"
  VR_ADCU_IPM_Obj_03_0x652/1(VR_ADCU_IPM_Obj_03_0x652FromOutData) -> VR_ADCU_IPM_Obj_03_0x652FromOutData/1  "VR_ADCU_IPM_Obj_03_0x652FromOutData"
  VR_ADCU_IPM_Obj_03_0x652FromInData/1 -> VR_ADCU_IPM_Obj_03_0x652/1(VR_ADCU_IPM_Obj_03_0x652FromInData)  "VR_ADCU_IPM_Obj_03_0x652FromInData"
  VR_ADCU_IPM_Obj_04_0x653/1(VR_ADCU_IPM_Obj_04_0x653FromOutData) -> VR_ADCU_IPM_Obj_04_0x653FromOutData/1  "VR_ADCU_IPM_Obj_04_0x653FromOutData"
  VR_ADCU_IPM_Obj_04_0x653FromInData/1 -> VR_ADCU_IPM_Obj_04_0x653/1(VR_ADCU_IPM_Obj_04_0x653FromInData)  "VR_ADCU_IPM_Obj_04_0x653FromInData"
  VR_ADCU_IPM_Obj_05_0x654/1(VR_ADCU_IPM_Obj_05_0x654FromOutData) -> VR_ADCU_IPM_Obj_05_0x654FromOutData/1  "VR_ADCU_IPM_Obj_05_0x654FromOutData"
  VR_ADCU_IPM_Obj_05_0x654FromInData/1 -> VR_ADCU_IPM_Obj_05_0x654/1(VR_ADCU_IPM_Obj_05_0x654FromInData)  "VR_ADCU_IPM_Obj_05_0x654FromInData"
  VR_ADCU_IPM_Obj_06_0x655/1(VR_ADCU_IPM_Obj_06_0x655FromOutData) -> VR_ADCU_IPM_Obj_06_0x655FromOutData/1  "VR_ADCU_IPM_Obj_06_0x655FromOutData"
  VR_ADCU_IPM_Obj_06_0x655FromInData/1 -> VR_ADCU_IPM_Obj_06_0x655/1(VR_ADCU_IPM_Obj_06_0x655FromInData)  "VR_ADCU_IPM_Obj_06_0x655FromInData"
  VR_ADCU_IPM_Obj_07_0x656/1(VR_ADCU_IPM_Obj_07_0x656FromOutData) -> VR_ADCU_IPM_Obj_07_0x656FromOutData/1  "VR_ADCU_IPM_Obj_07_0x656FromOutData"
  VR_ADCU_IPM_Obj_07_0x656FromInData/1 -> VR_ADCU_IPM_Obj_07_0x656/1(VR_ADCU_IPM_Obj_07_0x656FromInData)  "VR_ADCU_IPM_Obj_07_0x656FromInData"
  VR_ADCU_IPM_Obj_08_0x657/1(VR_ADCU_IPM_Obj_08_0x657FromOutData) -> VR_ADCU_IPM_Obj_08_0x657FromOutData/1  "VR_ADCU_IPM_Obj_08_0x657FromOutData"
  VR_ADCU_IPM_Obj_08_0x657FromInData/1 -> VR_ADCU_IPM_Obj_08_0x657/1(VR_ADCU_IPM_Obj_08_0x657FromInData)  "VR_ADCU_IPM_Obj_08_0x657FromInData"
  VR_ADCU_IPM_Obj_09_0x658/1(VR_ADCU_IPM_Obj_09_0x658FromOutData) -> VR_ADCU_IPM_Obj_09_0x658FromOutData/1  "VR_ADCU_IPM_Obj_09_0x658FromOutData"
  VR_ADCU_IPM_Obj_09_0x658FromInData/1 -> VR_ADCU_IPM_Obj_09_0x658/1(VR_ADCU_IPM_Obj_09_0x658FromInData)  "VR_ADCU_IPM_Obj_09_0x658FromInData"
  VR_ADCU_IPM_Obj_10_0x659/1(VR_ADCU_IPM_Obj_10_0x659FromOutData) -> VR_ADCU_IPM_Obj_10_0x659FromOutData/1  "VR_ADCU_IPM_Obj_10_0x659FromOutData"
  VR_ADCU_IPM_Obj_10_0x659FromInData/1 -> VR_ADCU_IPM_Obj_10_0x659/1(VR_ADCU_IPM_Obj_10_0x659FromInData)  "VR_ADCU_IPM_Obj_10_0x659FromInData"
  VR_ADCU_IPM_Obj_11_0x65A/1(VR_ADCU_IPM_Obj_11_0x65AFromOutData) -> VR_ADCU_IPM_Obj_11_0x65AFromOutData/1  "VR_ADCU_IPM_Obj_11_0x65AFromOutData"
  VR_ADCU_IPM_Obj_11_0x65AFromInData/1 -> VR_ADCU_IPM_Obj_11_0x65A/1(VR_ADCU_IPM_Obj_11_0x65AFromInData)  "VR_ADCU_IPM_Obj_11_0x65AFromInData"
  VR_ADCU_IPM_Obj_12_0x65B/1(VR_ADCU_IPM_Obj_12_0x65BFromOutData) -> VR_ADCU_IPM_Obj_12_0x65BFromOutData/1  "VR_ADCU_IPM_Obj_12_0x65BFromOutData"
  VR_ADCU_IPM_Obj_12_0x65BFromInData/1 -> VR_ADCU_IPM_Obj_12_0x65B/1(VR_ADCU_IPM_Obj_12_0x65BFromInData)  "VR_ADCU_IPM_Obj_12_0x65BFromInData"
  VR_ADCU_IPM_Obj_13_0x65C/1(VR_ADCU_IPM_Obj_13_0x65CFromOutData) -> VR_ADCU_IPM_Obj_13_0x65CFromOutData/1  "VR_ADCU_IPM_Obj_13_0x65CFromOutData"
  VR_ADCU_IPM_Obj_13_0x65CFromInData/1 -> VR_ADCU_IPM_Obj_13_0x65C/1(VR_ADCU_IPM_Obj_13_0x65CFromInData)  "VR_ADCU_IPM_Obj_13_0x65CFromInData"
  VR_ADCU_IPM_Obj_14_0x65D/1(VR_ADCU_IPM_Obj_14_0x65DFromOutData) -> VR_ADCU_IPM_Obj_14_0x65DFromOutData/1  "VR_ADCU_IPM_Obj_14_0x65DFromOutData"
  VR_ADCU_IPM_Obj_14_0x65DFromInData/1 -> VR_ADCU_IPM_Obj_14_0x65D/1(VR_ADCU_IPM_Obj_14_0x65DFromInData)  "VR_ADCU_IPM_Obj_14_0x65DFromInData"
  VR_ADCU_IPM_Obj_15_0x65E/1(VR_ADCU_IPM_Obj_15_0x65EFromOutData) -> VR_ADCU_IPM_Obj_15_0x65EFromOutData/1  "VR_ADCU_IPM_Obj_15_0x65EFromOutData"
  VR_ADCU_IPM_Obj_15_0x65EFromInData/1 -> VR_ADCU_IPM_Obj_15_0x65E/1(VR_ADCU_IPM_Obj_15_0x65EFromInData)  "VR_ADCU_IPM_Obj_15_0x65EFromInData"
  VR_ADCU_IPM_Obj_16_0x65F/1(VR_ADCU_IPM_Obj_16_0x65FFromOutData) -> VR_ADCU_IPM_Obj_16_0x65FFromOutData/1  "VR_ADCU_IPM_Obj_16_0x65FFromOutData"
  VR_ADCU_IPM_Obj_16_0x65FFromInData/1 -> VR_ADCU_IPM_Obj_16_0x65F/1(VR_ADCU_IPM_Obj_16_0x65FFromInData)  "VR_ADCU_IPM_Obj_16_0x65FFromInData"
  VR_ADCU_IPM_Obj_17_0x660/1(VR_ADCU_IPM_Obj_17_0x660FromOutData) -> VR_ADCU_IPM_Obj_17_0x660FromOutData/1  "VR_ADCU_IPM_Obj_17_0x660FromOutData"
  VR_ADCU_IPM_Obj_17_0x660FromInData/1 -> VR_ADCU_IPM_Obj_17_0x660/1(VR_ADCU_IPM_Obj_17_0x660FromInData)  "VR_ADCU_IPM_Obj_17_0x660FromInData"
  VR_ADCU_IPM_Obj_18_0x661/1(VR_ADCU_IPM_Obj_18_0x661FromOutData) -> VR_ADCU_IPM_Obj_18_0x661FromOutData/1  "VR_ADCU_IPM_Obj_18_0x661FromOutData"
  VR_ADCU_IPM_Obj_18_0x661FromInData/1 -> VR_ADCU_IPM_Obj_18_0x661/1(VR_ADCU_IPM_Obj_18_0x661FromInData)  "VR_ADCU_IPM_Obj_18_0x661FromInData"
  VR_ADCU_IPM_Obj_19_0x662/1(VR_ADCU_IPM_Obj_19_0x662FromOutData) -> VR_ADCU_IPM_Obj_19_0x662FromOutData/1  "VR_ADCU_IPM_Obj_19_0x662FromOutData"
  VR_ADCU_IPM_Obj_19_0x662FromInData/1 -> VR_ADCU_IPM_Obj_19_0x662/1(VR_ADCU_IPM_Obj_19_0x662FromInData)  "VR_ADCU_IPM_Obj_19_0x662FromInData"
  VR_ADCU_IPM_Obj_20_0x663/1(VR_ADCU_IPM_Obj_20_0x663FromOutData) -> VR_ADCU_IPM_Obj_20_0x663FromOutData/1  "VR_ADCU_IPM_Obj_20_0x663FromOutData"
  VR_ADCU_IPM_Obj_20_0x663FromInData/1 -> VR_ADCU_IPM_Obj_20_0x663/1(VR_ADCU_IPM_Obj_20_0x663FromInData)  "VR_ADCU_IPM_Obj_20_0x663FromInData"
  VR_ADCU_IPM_RightLine_0x590/1(VR_ADCU_IPM_RightLine_0x590FromOutData) -> VR_ADCU_IPM_RightLine_0x590FromOutData/1  "VR_ADCU_IPM_RightLine_0x590FromOutData"
  VR_ADCU_IPM_RightLine_0x590FromInData/1 -> VR_ADCU_IPM_RightLine_0x590/1(VR_ADCU_IPM_RightLine_0x590FromInData)  "VR_ADCU_IPM_RightLine_0x590FromInData"
  VR_ADCU_IPM_RightLine_0x591/1(VR_ADCU_IPM_RightLine_0x591FromOutData) -> VR_ADCU_IPM_RightLine_0x591FromOutData/1  "VR_ADCU_IPM_RightLine_0x591FromOutData"
  VR_ADCU_IPM_RightLine_0x591FromInData/1 -> VR_ADCU_IPM_RightLine_0x591/1(VR_ADCU_IPM_RightLine_0x591FromInData)  "VR_ADCU_IPM_RightLine_0x591FromInData"
  VR_ADCU_IPM_Traffic_01_0x670/1(VR_ADCU_IPM_Traffic_01_0x670FromOutData) -> VR_ADCU_IPM_Traffic_01_0x670FromOutData/1  "VR_ADCU_IPM_Traffic_01_0x670FromOutData"
  VR_ADCU_IPM_Traffic_01_0x670FromInData/1 -> VR_ADCU_IPM_Traffic_01_0x670/1(VR_ADCU_IPM_Traffic_01_0x670FromInData)  "VR_ADCU_IPM_Traffic_01_0x670FromInData"
  VR_ADCU_IPM_Traffic_02_0x671/1(VR_ADCU_IPM_Traffic_02_0x671FromOutData) -> VR_ADCU_IPM_Traffic_02_0x671FromOutData/1  "VR_ADCU_IPM_Traffic_02_0x671FromOutData"
  VR_ADCU_IPM_Traffic_02_0x671FromInData/1 -> VR_ADCU_IPM_Traffic_02_0x671/1(VR_ADCU_IPM_Traffic_02_0x671FromInData)  "VR_ADCU_IPM_Traffic_02_0x671FromInData"
  VR_ADCU_IPM_Traffic_03_0x672/1(VR_ADCU_IPM_Traffic_03_0x672FromOutData) -> VR_ADCU_IPM_Traffic_03_0x672FromOutData/1  "VR_ADCU_IPM_Traffic_03_0x672FromOutData"
  VR_ADCU_IPM_Traffic_03_0x672FromInData/1 -> VR_ADCU_IPM_Traffic_03_0x672/1(VR_ADCU_IPM_Traffic_03_0x672FromInData)  "VR_ADCU_IPM_Traffic_03_0x672FromInData"
  VR_ADCU_IPM_Traffic_04_0x673/1(VR_ADCU_IPM_Traffic_04_0x673FromOutData) -> VR_ADCU_IPM_Traffic_04_0x673FromOutData/1  "VR_ADCU_IPM_Traffic_04_0x673FromOutData"
  VR_ADCU_IPM_Traffic_04_0x673FromInData/1 -> VR_ADCU_IPM_Traffic_04_0x673/1(VR_ADCU_IPM_Traffic_04_0x673FromInData)  "VR_ADCU_IPM_Traffic_04_0x673FromInData"
  VR_ADCU_IPM_Traffic_05_0x674/1(VR_ADCU_IPM_Traffic_05_0x674FromOutData) -> VR_ADCU_IPM_Traffic_05_0x674FromOutData/1  "VR_ADCU_IPM_Traffic_05_0x674FromOutData"
  VR_ADCU_IPM_Traffic_05_0x674FromInData/1 -> VR_ADCU_IPM_Traffic_05_0x674/1(VR_ADCU_IPM_Traffic_05_0x674FromInData)  "VR_ADCU_IPM_Traffic_05_0x674FromInData"
  VR_ADCU_IPM_Traffic_06_0x675/1(VR_ADCU_IPM_Traffic_06_0x675FromOutData) -> VR_ADCU_IPM_Traffic_06_0x675FromOutData/1  "VR_ADCU_IPM_Traffic_06_0x675FromOutData"
  VR_ADCU_IPM_Traffic_06_0x675FromInData/1 -> VR_ADCU_IPM_Traffic_06_0x675/1(VR_ADCU_IPM_Traffic_06_0x675FromInData)  "VR_ADCU_IPM_Traffic_06_0x675FromInData"
  VR_ADCU_IPM_VLC_0x393/1(VR_ADCU_IPM_VLC_0x393FromOutData) -> VR_ADCU_IPM_VLC_0x393FromOutData/1  "VR_ADCU_IPM_VLC_0x393FromOutData"
  VR_ADCU_IPM_VLC_0x393FromInData/1 -> VR_ADCU_IPM_VLC_0x393/1(VR_ADCU_IPM_VLC_0x393FromInData)  "VR_ADCU_IPM_VLC_0x393FromInData"
  VR_ADCU_MRR_0x338/1(VR_ADCU_MRR_0x338FromOutData) -> VR_ADCU_MRR_0x338FromOutData/1  "VR_ADCU_MRR_0x338FromOutData"
  VR_ADCU_MRR_0x338FromInData/1 -> VR_ADCU_MRR_0x338/1(VR_ADCU_MRR_0x338FromInData)  "VR_ADCU_MRR_0x338FromInData"
  VR_ADCU_MRR_0x339/1(VR_ADCU_MRR_0x339FromOutData) -> VR_ADCU_MRR_0x339FromOutData/1  "VR_ADCU_MRR_0x339FromOutData"
  VR_ADCU_MRR_0x339FromInData/1 -> VR_ADCU_MRR_0x339/1(VR_ADCU_MRR_0x339FromInData)  "VR_ADCU_MRR_0x339FromInData"
  VR_ADCU_MRR_0x346/1(VR_ADCU_MRR_0x346FromOutData) -> VR_ADCU_MRR_0x346FromOutData/1  "VR_ADCU_MRR_0x346FromOutData"
  VR_ADCU_MRR_0x346FromInData/1 -> VR_ADCU_MRR_0x346/1(VR_ADCU_MRR_0x346FromInData)  "VR_ADCU_MRR_0x346FromInData"
  VR_ADCU_MRR_FRObj_0x379/1(VR_ADCU_MRR_FRObj_0x379FromOutData) -> VR_ADCU_MRR_FRObj_0x379FromOutData/1  "VR_ADCU_MRR_FRObj_0x379FromOutData"
  VR_ADCU_MRR_FRObj_0x379FromInData/1 -> VR_ADCU_MRR_FRObj_0x379/1(VR_ADCU_MRR_FRObj_0x379FromInData)  "VR_ADCU_MRR_FRObj_0x379FromInData"
  VR_ADCU_MRR_LRObj_0x580/1(VR_ADCU_MRR_LRObj_0x580FromOutData) -> VR_ADCU_MRR_LRObj_0x580FromOutData/1  "VR_ADCU_MRR_LRObj_0x580FromOutData"
  VR_ADCU_MRR_LRObj_0x580FromInData/1 -> VR_ADCU_MRR_LRObj_0x580/1(VR_ADCU_MRR_LRObj_0x580FromInData)  "VR_ADCU_MRR_LRObj_0x580FromInData"
  VR_ADCU_MRR_ObjHeader_0x680/1(VR_ADCU_MRR_ObjHeader_0x680FromOutData) -> VR_ADCU_MRR_ObjHeader_0x680FromOutData/1  "VR_ADCU_MRR_ObjHeader_0x680FromOutData"
  VR_ADCU_MRR_ObjHeader_0x680FromInData/1 -> VR_ADCU_MRR_ObjHeader_0x680/1(VR_ADCU_MRR_ObjHeader_0x680FromInData)  "VR_ADCU_MRR_ObjHeader_0x680FromInData"
  VR_ADCU_MRR_Obj_01_02_0x690FromInData/1 -> VR_ADCU_MRR_Obj_01_02_0x690/1(VR_ADCU_MRR_Obj_01_02_0x690FromInData)  "VR_ADCU_MRR_Obj_01_02_0x690FromInData"
  VR_ADCU_MRR_Obj_03_04_0x691/1(VR_ADCU_MRR_Obj_03_04_0x691FromOutData) -> VR_ADCU_MRR_Obj_03_04_0x691FromOutData/1  "VR_ADCU_MRR_Obj_03_04_0x691FromOutData"
  VR_ADCU_MRR_Obj_03_04_0x691FromInData/1 -> VR_ADCU_MRR_Obj_03_04_0x691/1(VR_ADCU_MRR_Obj_03_04_0x691FromInData)  "VR_ADCU_MRR_Obj_03_04_0x691FromInData"
  VR_ADCU_MRR_Obj_05_06_0x692/1(VR_ADCU_MRR_Obj_05_06_0x692FromOutData) -> VR_ADCU_MRR_Obj_05_06_0x692FromOutData/1  "VR_ADCU_MRR_Obj_05_06_0x692FromOutData"
  VR_ADCU_MRR_Obj_05_06_0x692FromInData/1 -> VR_ADCU_MRR_Obj_05_06_0x692/1(VR_ADCU_MRR_Obj_05_06_0x692FromInData)  "VR_ADCU_MRR_Obj_05_06_0x692FromInData"
  VR_ADCU_MRR_Obj_07_08_0x693/1(VR_ADCU_MRR_Obj_07_08_0x693FromOutData) -> VR_ADCU_MRR_Obj_07_08_0x693FromOutData/1  "VR_ADCU_MRR_Obj_07_08_0x693FromOutData"
  VR_ADCU_MRR_Obj_07_08_0x693FromInData/1 -> VR_ADCU_MRR_Obj_07_08_0x693/1(VR_ADCU_MRR_Obj_07_08_0x693FromInData)  "VR_ADCU_MRR_Obj_07_08_0x693FromInData"
  VR_ADCU_MRR_Obj_09_10_0x694/1(VR_ADCU_MRR_Obj_09_10_0x694FromOutData) -> VR_ADCU_MRR_Obj_09_10_0x694FromOutData/1  "VR_ADCU_MRR_Obj_09_10_0x694FromOutData"
  VR_ADCU_MRR_Obj_09_10_0x694FromInData/1 -> VR_ADCU_MRR_Obj_09_10_0x694/1(VR_ADCU_MRR_Obj_09_10_0x694FromInData)  "VR_ADCU_MRR_Obj_09_10_0x694FromInData"
  VR_ADCU_MRR_Obj_11_12_0x695/1(VR_ADCU_MRR_Obj_11_12_0x695FromOutData) -> VR_ADCU_MRR_Obj_11_12_0x695FromOutData/1  "VR_ADCU_MRR_Obj_11_12_0x695FromOutData"
  VR_ADCU_MRR_Obj_11_12_0x695FromInData/1 -> VR_ADCU_MRR_Obj_11_12_0x695/1(VR_ADCU_MRR_Obj_11_12_0x695FromInData)  "VR_ADCU_MRR_Obj_11_12_0x695FromInData"
  VR_ADCU_MRR_Obj_13_14_0x696/1(VR_ADCU_MRR_Obj_13_14_0x696FromOutData) -> VR_ADCU_MRR_Obj_13_14_0x696FromOutData/1  "VR_ADCU_MRR_Obj_13_14_0x696FromOutData"
  VR_ADCU_MRR_Obj_13_14_0x696FromInData/1 -> VR_ADCU_MRR_Obj_13_14_0x696/1(VR_ADCU_MRR_Obj_13_14_0x696FromInData)  "VR_ADCU_MRR_Obj_13_14_0x696FromInData"
  VR_ADCU_MRR_Obj_15_16_0x697/1(VR_ADCU_MRR_Obj_15_16_0x697FromOutData) -> VR_ADCU_MRR_Obj_15_16_0x697FromOutData/1  "VR_ADCU_MRR_Obj_15_16_0x697FromOutData"
  VR_ADCU_MRR_Obj_15_16_0x697FromInData/1 -> VR_ADCU_MRR_Obj_15_16_0x697/1(VR_ADCU_MRR_Obj_15_16_0x697FromInData)  "VR_ADCU_MRR_Obj_15_16_0x697FromInData"
  VR_ADCU_MRR_Obj_17_18_0x698/1(VR_ADCU_MRR_Obj_17_18_0x698FromOutData) -> VR_ADCU_MRR_Obj_17_18_0x698FromOutData/1  "VR_ADCU_MRR_Obj_17_18_0x698FromOutData"
  VR_ADCU_MRR_Obj_17_18_0x698FromInData/1 -> VR_ADCU_MRR_Obj_17_18_0x698/1(VR_ADCU_MRR_Obj_17_18_0x698FromInData)  "VR_ADCU_MRR_Obj_17_18_0x698FromInData"
  VR_ADCU_MRR_Obj_19_20_0x699/1(VR_ADCU_MRR_Obj_19_20_0x699FromOutData) -> VR_ADCU_MRR_Obj_19_20_0x699FromOutData/1  "VR_ADCU_MRR_Obj_19_20_0x699FromOutData"
  VR_ADCU_MRR_Obj_19_20_0x699FromInData/1 -> VR_ADCU_MRR_Obj_19_20_0x699/1(VR_ADCU_MRR_Obj_19_20_0x699FromInData)  "VR_ADCU_MRR_Obj_19_20_0x699FromInData"
  VR_ADCU_MRR_Obj_21_22_0x69A/1(VR_ADCU_MRR_Obj_21_22_0x69AFromOutData) -> VR_ADCU_MRR_Obj_21_22_0x69AFromOutData/1  "VR_ADCU_MRR_Obj_21_22_0x69AFromOutData"
  VR_ADCU_MRR_Obj_21_22_0x69AFromInData/1 -> VR_ADCU_MRR_Obj_21_22_0x69A/1(VR_ADCU_MRR_Obj_21_22_0x69AFromInData)  "VR_ADCU_MRR_Obj_21_22_0x69AFromInData"
  VR_ADCU_MRR_Obj_23_24_0x69B/1(VR_ADCU_MRR_Obj_23_24_0x69BFromOutData) -> VR_ADCU_MRR_Obj_23_24_0x69BFromOutData/1  "VR_ADCU_MRR_Obj_23_24_0x69BFromOutData"
  VR_ADCU_MRR_Obj_23_24_0x69BFromInData/1 -> VR_ADCU_MRR_Obj_23_24_0x69B/1(VR_ADCU_MRR_Obj_23_24_0x69BFromInData)  "VR_ADCU_MRR_Obj_23_24_0x69BFromInData"
  VR_ADCU_MRR_Obj_25_26_0x69C/1(VR_ADCU_MRR_Obj_25_26_0x69CFromOutData) -> VR_ADCU_MRR_Obj_25_26_0x69CFromOutData/1  "VR_ADCU_MRR_Obj_25_26_0x69CFromOutData"
  VR_ADCU_MRR_Obj_25_26_0x69CFromInData/1 -> VR_ADCU_MRR_Obj_25_26_0x69C/1(VR_ADCU_MRR_Obj_25_26_0x69CFromInData)  "VR_ADCU_MRR_Obj_25_26_0x69CFromInData"
  VR_ADCU_MRR_Obj_27_28_0x69D/1(VR_ADCU_MRR_Obj_27_28_0x69DFromOutData) -> VR_ADCU_MRR_Obj_27_28_0x69DFromOutData/1  "VR_ADCU_MRR_Obj_27_28_0x69DFromOutData"
  VR_ADCU_MRR_Obj_27_28_0x69DFromInData/1 -> VR_ADCU_MRR_Obj_27_28_0x69D/1(VR_ADCU_MRR_Obj_27_28_0x69DFromInData)  "VR_ADCU_MRR_Obj_27_28_0x69DFromInData"
  VR_ADCU_MRR_Obj_29_30_0x69E/1(VR_ADCU_MRR_Obj_29_30_0x69EFromOutData) -> VR_ADCU_MRR_Obj_29_30_0x69EFromOutData/1  "VR_ADCU_MRR_Obj_29_30_0x69EFromOutData"
  VR_ADCU_MRR_Obj_29_30_0x69EFromInData/1 -> VR_ADCU_MRR_Obj_29_30_0x69E/1(VR_ADCU_MRR_Obj_29_30_0x69EFromInData)  "VR_ADCU_MRR_Obj_29_30_0x69EFromInData"
  VR_ADCU_MRR_Obj_31_32_0x69F/1(VR_ADCU_MRR_Obj_31_32_0x69FFromOutData) -> VR_ADCU_MRR_Obj_31_32_0x69FFromOutData/1  "VR_ADCU_MRR_Obj_31_32_0x69FFromOutData"
  VR_ADCU_MRR_Obj_31_32_0x69FFromInData/1 -> VR_ADCU_MRR_Obj_31_32_0x69F/1(VR_ADCU_MRR_Obj_31_32_0x69FFromInData)  "VR_ADCU_MRR_Obj_31_32_0x69FFromInData"
  VR_ADCU_MRR_Obj_01_02_0x690/1(VR_ADCU_MRR_Obj_01_02_0x690FromOutData) -> VR_ADCU_MRR_Obj_01_02_0x690FromOutData/1  "VR_ADCU_MRR_Obj_01_02_0x690FromOutData"
